simulink model "OMNI_BOT_MOEDL2"  (R2024b)
settings: Solver=VariableStepAuto  StartTime=0.0  StopTime=300  RelTol=1e-3
settings Model: Creator=PC  LastModifiedBy=Admin
settings SolverCC: AlgebraicLoopSolver=TrustRegion
settings DebuggingCC: UnconnectedInputMsg=warning  UnconnectedOutputMsg=warning  UnconnectedLineMsg=warning
settings ModelReferenceCC: EnableRefExpFcnMdlSchedulingChecks=on
settings SFSimCC: CustomCodeUndefinedFunction=UseInterfaceOnly
settings RTWCC: GPUComputeCapability=3.5

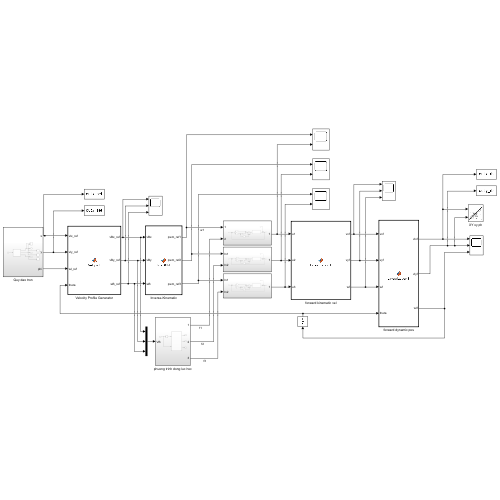
[thumbnail: Simulink's stored preview of the top-level diagram]
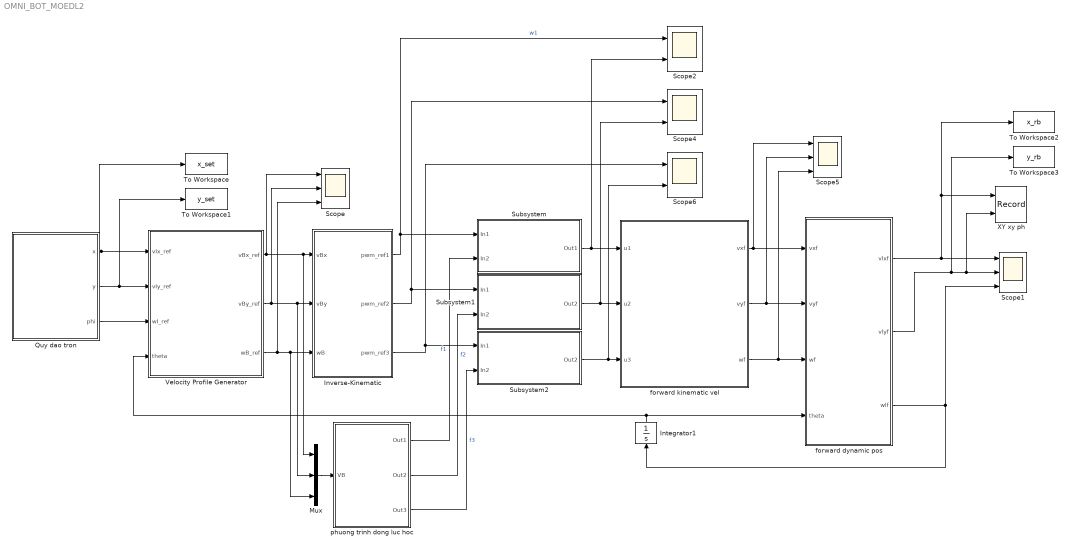
== system OMNI_BOT_MOEDL2 ==
  Integrator1 : Integrator
  Inverse-Kinematic : MATLAB Function  TreatAsAtomicUnit=on
  Mux : Mux  Inputs=3
  Quy dao tron : Subsystem
  Scope : Scope  NumInputPorts=3
  Scope1 : Scope  NumInputPorts=3
  Scope2 : Scope  NumInputPorts=2
  Scope4 : Scope  NumInputPorts=2
  Scope5 : Scope  NumInputPorts=3
  Scope6 : Scope  NumInputPorts=2
  Subsystem : Subsystem
  Subsystem1 : Subsystem
  Subsystem2 : Subsystem
  To Workspace : ToWorkspace  VariableName=x_set  SaveFormat=Timeseries  SampleTime=-1
  To Workspace1 : ToWorkspace  VariableName=y_set  SaveFormat=Timeseries  SampleTime=-1
  To Workspace2 : ToWorkspace  VariableName=x_rb  SaveFormat=Timeseries  SampleTime=-1
  To Workspace3 : ToWorkspace  VariableName=y_rb  SaveFormat=Timeseries  SampleTime=-1
  Velocity Profile Generator : MATLAB Function  TreatAsAtomicUnit=on
  XY xy ph : Record  FileSettingsInternal="{\"entries\":[{\"content\":{\"excelSettings\":{\"content\":{},\"type\":\"Streamout.ExcelSettings\"}},\"type\":\"Streamout.FileSettingStorage\",\"uuid\":\"\"}],\"packageUris\":[\"http:\\/\\/schema.mathworks.com\\/mf0\\/streamout_blocks\\/R2020a\"],\"version\":\"1.0\"}"  Layout=[1 1]  SignalsInternal="{\"entries\":[{\"content\":{\"signals\":[{\"content\":{\"blockPath\":[],\"dimensions\":[1],\"domain\":\"\",\"lineColor\":\"#a2142f\",\"plots\":[ 1 ],\"port\":1,\"signalID\":1,\"signalName\":\"forward dynamic pos:1\"},\"type\":\"RecordBlkView.Signal\",\"uuid\":\"\"},{\"content\":{\"blockPath\":[],\"dimensions\":[1],\"domain\":\"\",\"lineColor\":\"#139fff\",\"plots\":[ 1 ],\"port\":2,\"signalID\":2,\"signalName\":\"forward dynamic pos:2\"},\"type\":\"RecordBlkView.Signal\",\"uuid\":\"\"}]},\"type\":\"RecordBlkView.InputSignals\",\"uuid\":\"\"}],\"packageUris\":[\"http:\\/\\/schema.mathworks.com\\/mf0\\/streamout_blocks\\/R2020a\"],\"version\":\"1.0\"}"  VisualizationBindings="{\"xyplotplugin\":{\"info\":[{\"series\":[{\"bindingParametersList\":[{\"parameter\":\"X-Axis\",\"signalID\":1,\"signalName\":\"forward dynamic pos:1\"},{\"parameter\":\"Y-Axis\",\"signalID\":2,\"signalName\":\"forward dynamic pos:2\"}],\"seriesID\":0}],\"subplotID\":1}]}}"  CompatibilityTag=XY  st=-1
  forward dynamic pos : MATLAB Function  TreatAsAtomicUnit=on
  forward kinematic vel : MATLAB Function  TreatAsAtomicUnit=on
  phuong trinh dong luc hoc : Subsystem
  wires:
  Velocity Profile Generator/1(vBx_ref) -> Mux/1, Inverse-Kinematic/1(vBx), Scope/1
  Velocity Profile Generator/2(vBy_ref) -> Mux/2, Inverse-Kinematic/2(vBy), Scope/2
  Velocity Profile Generator/3(wB_ref) -> Mux/3, Inverse-Kinematic/3(wB), Scope/3
  Quy dao tron/1(x) -> To Workspace/1, Velocity Profile Generator/1(vIx_ref)
  Quy dao tron/2(y) -> To Workspace1/1, Velocity Profile Generator/2(vIy_ref)
  Quy dao tron/3(phi) -> Velocity Profile Generator/3(wI_ref)
  Inverse-Kinematic/1(pwm_ref1) -> Scope2/1, Subsystem/1(In1)  "w1"
  Inverse-Kinematic/2(pwm_ref2) -> Scope4/1, Subsystem1/1("In1 ")
  Inverse-Kinematic/3(pwm_ref3) -> Scope6/1, Subsystem2/1("In1 ")
  Subsystem/1(Out1) -> Scope2/2, forward kinematic vel/1(u1)
  Subsystem2/1(Out2) -> Scope6/2, forward kinematic vel/3(u3)
  Subsystem1/1(Out2) -> Scope4/2, forward kinematic vel/2(u2)
  forward dynamic pos/1(vlxf) -> To Workspace2/1, XY xy ph/1, Scope1/1
  forward kinematic vel/1(vxf) -> Scope5/1, forward dynamic pos/1(vxf)
  forward kinematic vel/2(vyf) -> Scope5/2, forward dynamic pos/2(vyf)
  forward kinematic vel/3(wf) -> Scope5/3, forward dynamic pos/3(wf)
  forward dynamic pos/3(wlf) -> Scope1/3, Integrator1/1
  forward dynamic pos/2(vlyf) -> To Workspace3/1, XY xy ph/2, Scope1/2
  Integrator1/1 -> forward dynamic pos/4(theta), Velocity Profile Generator/4(theta)
  phuong trinh dong luc hoc/1(Out1) -> Subsystem/2(In2)  "f1"
  phuong trinh dong luc hoc/2(Out2) -> Subsystem1/2("In2 ")  "f2"
  phuong trinh dong luc hoc/3(Out3) -> Subsystem2/2("In2 ")  "f3"
  Mux/1 -> phuong trinh dong luc hoc/1(VB)

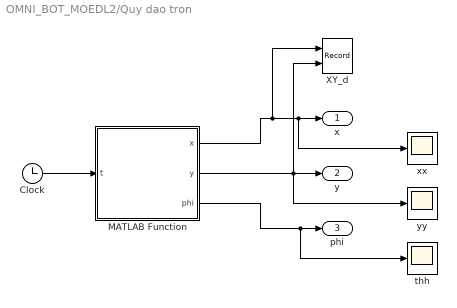
== system OMNI_BOT_MOEDL2/Quy dao tron ==
  Clock : Clock
  MATLAB Function : MATLAB Function  TreatAsAtomicUnit=on
  XY_d : Record  FileSettingsInternal="{\"entries\":[{\"content\":{\"excelSettings\":{\"content\":{},\"type\":\"Streamout.ExcelSettings\"}},\"type\":\"Streamout.FileSettingStorage\",\"uuid\":\"\"}],\"packageUris\":[\"http:\\/\\/schema.mathworks.com\\/mf0\\/streamout_blocks\\/R2020a\"],\"version\":\"1.0\"}"  Layout=[1 1]  SignalsInternal="{\"entries\":[{\"content\":{\"signals\":[{\"content\":{\"blockPath\":[],\"dimensions\":[1],\"domain\":\"\",\"lineColor\":\"#a2142f\",\"plots\":[ 1 ],\"port\":1,\"signalID\":1,\"signalName\":\"MATLAB Function:1\"},\"type\":\"RecordBlkView.Signal\",\"uuid\":\"\"},{\"content\":{\"blockPath\":[],\"dimensions\":[1],\"domain\":\"\",\"lineColor\":\"#139fff\",\"plots\":[ 1 ],\"port\":2,\"signalID\":2,\"signalName\":\"MATLAB Function:2\"},\"type\":\"RecordBlkView.Signal\",\"uuid\":\"\"}]},\"type\":\"RecordBlkView.InputSignals\",\"uuid\":\"\"}],\"packageUris\":[\"http:\\/\\/schema.mathworks.com\\/mf0\\/streamout_blocks\\/R2020a\"],\"version\":\"1.0\"}"  VisualizationBindings="{\"xyplotplugin\":{\"info\":[{\"series\":[{\"bindingParametersList\":[{\"parameter\":\"X-Axis\",\"signalID\":1,\"signalName\":\"MATLAB Function:1\"},{\"parameter\":\"Y-Axis\",\"signalID\":2,\"signalName\":\"MATLAB Function:2\"}],\"seriesID\":0}],\"subplotID\":1}]}}"  CompatibilityTag=XY  st=0
  thh : Scope
  xx : Scope
  yy : Scope
  x : Outport
  y : Outport  Port=2
  phi : Outport  Port=3
  wires:
  Clock/1 -> MATLAB Function/1(t)
  MATLAB Function/1(x) -> XY_d/1, xx/1, x/1
  MATLAB Function/2(y) -> yy/1, XY_d/2, y/1
  MATLAB Function/3(phi) -> thh/1, phi/1

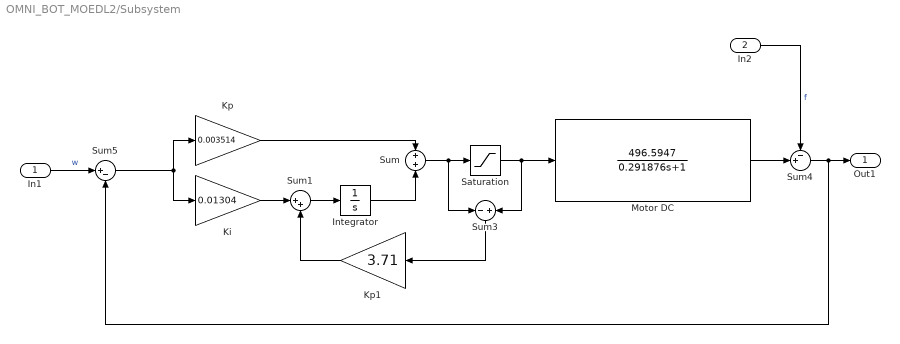
== system OMNI_BOT_MOEDL2/Subsystem ==
  In1 : Inport
  In2 : Inport  Port=2
  Integrator : Integrator
  Ki : Gain  Gain=0.01304
  Kp : Gain  Gain=0.003514
  Kp1 : Gain  Gain=3.71
  Motor DC : TransferFcn  Numerator=[496.5947]  Denominator=[0.291876 1]
  Saturation : Saturate  UpperLimit=12  LowerLimit=-12
  Sum : Sum  Inputs=+|+
  Sum1 : Sum  Inputs=|++
  Sum3 : Sum  Inputs=-|+
  Sum4 : Sum  Inputs=-+|
  Sum5 : Sum  Inputs=|+-
  Out1 : Outport  VectorParamsAs1DForOutWhenUnconnected=off
  wires:
  Integrator/1 -> Sum/2
  Sum1/1 -> Integrator/1
  Sum5/1 -> Kp/1, Ki/1
  Sum3/1 -> Kp1/1
  Kp/1 -> Sum/1
  Sum/1 -> Sum3/1, Saturation/1
  In1/1 -> Sum5/1  "w"
  Motor DC/1 -> Sum4/2
  Kp1/1 -> Sum1/2
  In2/1 -> Sum4/1  "f"
  Sum4/1 -> Out1/1, Sum5/2
  Ki/1 -> Sum1/1
  Saturation/1 -> Motor DC/1, Sum3/2

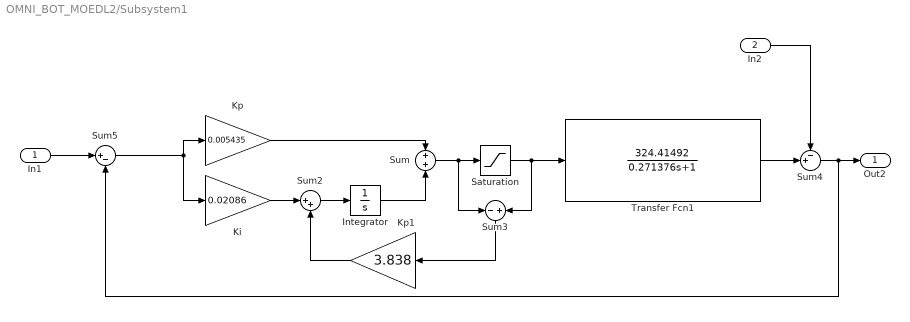
== system OMNI_BOT_MOEDL2/Subsystem1 ==
  "In1 " : Inport
  "In2 " : Inport  Port=2
  Integrator : Integrator
  Ki : Gain  Gain=0.02086
  Kp : Gain  Gain=0.005435
  Kp1 : Gain  Gain=3.838
  Saturation : Saturate  UpperLimit=12  LowerLimit=-12
  Sum : Sum  Inputs=+|+
  Sum2 : Sum  Inputs=|++
  Sum3 : Sum  Inputs=-|+
  Sum4 : Sum  Inputs=-+|
  Sum5 : Sum  Inputs=|+-
  Transfer Fcn1 : TransferFcn  Numerator=[324.41492]  Denominator=[0.271376 1]
  Out2 : Outport  VectorParamsAs1DForOutWhenUnconnected=off
  wires:
  "In2 "/1 -> Sum4/1
  Ki/1 -> Sum2/1
  Kp1/1 -> Sum2/2
  Transfer Fcn1/1 -> Sum4/2
  Sum/1 -> Sum3/1, Saturation/1
  Sum3/1 -> Kp1/1
  Kp/1 -> Sum/1
  Sum4/1 -> Out2/1, Sum5/2
  Sum2/1 -> Integrator/1
  Sum5/1 -> Kp/1, Ki/1
  Integrator/1 -> Sum/2
  "In1 "/1 -> Sum5/1
  Saturation/1 -> Transfer Fcn1/1, Sum3/2

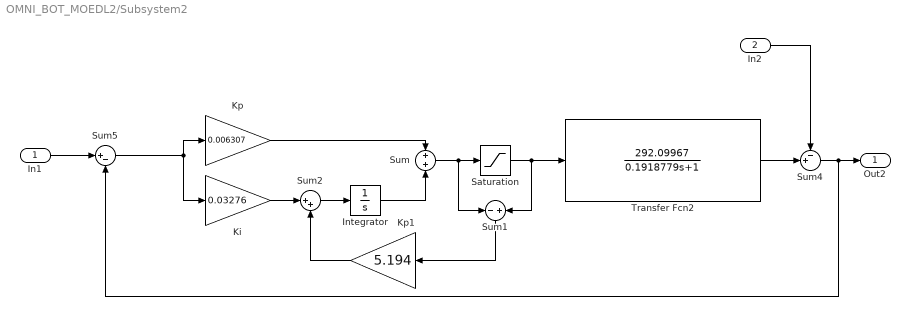
== system OMNI_BOT_MOEDL2/Subsystem2 ==
  "In1 " : Inport
  "In2 " : Inport  Port=2
  Integrator : Integrator
  Ki : Gain  Gain=0.03276
  Kp : Gain  Gain=0.006307
  Kp1 : Gain  Gain=5.194
  Saturation : Saturate  UpperLimit=12  LowerLimit=-12
  Sum : Sum  Inputs=+|+
  Sum1 : Sum  Inputs=-|+
  Sum2 : Sum  Inputs=|++
  Sum4 : Sum  Inputs=-+|
  Sum5 : Sum  Inputs=|+-
  Transfer Fcn2 : TransferFcn  Numerator=[292.09967]  Denominator=[0.1918779 1]
  Out2 : Outport  VectorParamsAs1DForOutWhenUnconnected=off
  wires:
  Transfer Fcn2/1 -> Sum4/2
  Integrator/1 -> Sum/2
  Sum2/1 -> Integrator/1
  Sum5/1 -> Kp/1, Ki/1
  Ki/1 -> Sum2/1
  "In2 "/1 -> Sum4/1
  Sum4/1 -> Out2/1, Sum5/2
  Kp1/1 -> Sum2/2
  Kp/1 -> Sum/1
  Sum1/1 -> Kp1/1
  Saturation/1 -> Transfer Fcn2/1, Sum1/2
  Sum/1 -> Sum1/1, Saturation/1
  "In1 "/1 -> Sum5/1

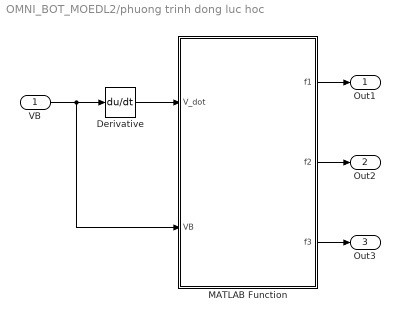
== system OMNI_BOT_MOEDL2/phuong trinh dong luc hoc ==
  VB : Inport
  Derivative : Derivative
  MATLAB Function : MATLAB Function  TreatAsAtomicUnit=on
  Out1 : Outport  VectorParamsAs1DForOutWhenUnconnected=off
  Out2 : Outport  Port=2  VectorParamsAs1DForOutWhenUnconnected=off
  Out3 : Outport  Port=3  VectorParamsAs1DForOutWhenUnconnected=off
  wires:
  MATLAB Function/3(f3) -> Out3/1
  MATLAB Function/2(f2) -> Out2/1
  MATLAB Function/1(f1) -> Out1/1
  Derivative/1 -> MATLAB Function/1(V_dot)
  VB/1 -> MATLAB Function/2(VB), Derivative/1

== matlab function OMNI_BOT_MOEDL2/phuong trinh dong luc hoc/MATLAB Function ==
  data: V_dot input; f1 output; VB input; f2 output; f3 output
function [f1,f2,f3] = fcn(V_dot,VB)
m = 4; % Mass of the mobile robot
Jz = 0.5; % Moment of inertia of the robot
N=56; % Reduction Ratio of the motors (adimensional)
eta=1; % Mechanical coupling efficiency (adimensional)
l=0.137;  % % Distance between base center and wheel center [m]
rw=0.0259; % Radius of wheels [m]

B2 = [-cos(pi/6) -cos(pi/3) rw;
      cos(pi/6) -cos(pi/3) rw;
      0 1 rw];

H1 = [1/m 0 0;
      0 1/m 0;
      0 0 1/Jz];
 
F1 =inv(B2)*inv(H1)*(-VB + V_dot);

f1 = F1(1,:);
f2 = F1(2,:);
f3 = F1(3,:);
end

== matlab function OMNI_BOT_MOEDL2/forward dynamic pos ==
  data: vlxf output; vlyf output; wlf output; vxf input; vyf input; wf input; theta input
function [vlxf,vlyf,wlf] = Linearization3(vxf,vyf,wf,theta)
%Dong hoc nghich tim vi tri

N=56; % Reduction Ratio of the motors (adimensional)
eta=1; % Mechanical coupling efficiency (adimensional)
l=0.137;  % % Distance between base center and wheel center [m]
rw=0.0259; % Radius of wheels [m]

B = [-cos(pi/6) -cos(pi/3) rw;
     cos(pi/6) -cos(pi/3) rw;
     0 1 rw];

A1 = [cosd(theta) -sind(theta) 0; sind(theta) cosd(theta) 0; 0 0 1];

vel = A1*[vxf;vyf;wf];

 vlxf = vel(1,:);
 vlyf = vel(2,:);
 wlf = vel(3,:);
end

== matlab function OMNI_BOT_MOEDL2/forward kinematic vel ==
  data: vxf output; vyf output; wf output; u1 input; u2 input; u3 input
function [vxf,vyf,wf] = Linearization1(u1,u2,u3)
%Dong hoc nghich tim van toc

N=56; % Reduction Ratio of the motors (adimensional)
eta=1; % Mechanical coupling efficiency (adimensional)
l=0.137;  % % Distance between base center and wheel center [m]
rw=0.0259; % Radius of wheels [m]

 A2 = [-cos(pi/6) -cos(pi/3) rw;
     cos(pi/6) -cos(pi/3) rw;
     0 1 rw];
 
 vel = (rw/N)*inv(A2)*[u1;u2;u3];
 vxf = vel(1,:);
 vyf = vel(2,:);
 wf = vel(3,:);
end

== matlab function OMNI_BOT_MOEDL2/Inverse-Kinematic ==
  data: vBx input; pwm_ref1 output; vBy input; wB input; pwm_ref2 output; pwm_ref3 output
function [pwm_ref1,pwm_ref2,pwm_ref3] = Inv_KIN(vBx,vBy,wB)

% Tu huong va goc quay dong co tinh ra van toc goc 3 dong co (pwm cua 3
% dong co)

N=56; % Reduction Ratio of the motors (adimensional)
eta=1; % Mechanical coupling efficiency (adimensional)
l=0.137;  % % Distance between base center and wheel center [m]
rw=0.0259; % Radius of wheels [m]

B = [-cos(pi/6) -cos(pi/3) rw;
     cos(pi/6) -cos(pi/3) rw;
     0 1 rw];
W=(N/rw)*B*[vBx;vBy;wB];

pwm_ref1=W(1,:); % Angular speed of motor 1 (reference value)
pwm_ref2=W(2,:); % Angular speed of motor 2 (reference value)
pwm_ref3=W(3,:); % Angular speed of motor 3 (reference value)
end

== matlab function OMNI_BOT_MOEDL2/Velocity Profile Generator ==
  data: vIx_ref input; vBx_ref output; vIy_ref input; wI_ref input; vBy_ref output; wB_ref output; theta input
function [vBx_ref,vBy_ref,wB_ref] = Vel_prof(vIx_ref,vIy_ref,wI_ref,theta)
% Huong va goc quay dong co

N=56; % Reduction Ratio of the motors (adimensional)
eta=1; % Mechanical coupling efficiency (adimensional)
l=0.137;  % Distance between base center and wheel center [m]
rw=0.0259; % Wheel radius [m]

A=[cosd(theta) -sind(theta) 0; sind(theta) cosd(theta) 0; 0 0 1];

vel1 = A\[vIx_ref;vIy_ref;wI_ref]; 


vBx_ref=vel1(1,:);% linear velocity along x-direction  [BODY-FRAME]
vBy_ref=vel1(2,:);% linear velocity along y-direction  [BODY-FRAME]
wB_ref=vel1(3,:); % Angular velocity around z-axis     [BODY-FRAME]
end

== matlab function OMNI_BOT_MOEDL2/Quy dao tron/MATLAB Function ==
  data: x output; t input; y output; phi output
function [x,y,phi] = fcn(t)
x=1.*cos((pi/50).*t);
y=1.*sin((pi/50).*t);
phi=(pi/50).*t + pi/2;
end
